simulink model "Tank_Modell_Student_2_tank_RL"  (R2020b)
settings: Solver=ode45  StartTime=0.0  StopTime=1200  RelTol=1e-3
values from neighbouring files (symbols this model uses):
  D = [0]    [Spielwiese.m]    (also in set_parameter.m; set_parameter_2_tank.m; set_parameter_3_tank.m)
undefined symbols (not defined in the file or in its folder): parRateLim, parReg, parSys
settings Model: Creator=Wolfgang Kemmetmüller  LastModifiedBy=simon
settings DataIOCC: LimitDataPoints=on  SaveFormat=Array  ReturnWorkspaceOutputs=off
settings OptimizationCC: BlockReduction=off  BooleanDataType=off  LifeSpan=inf
settings DebuggingCC: SaveWithParameterizedLinksMsg=none  UnderspecifiedInitializationDetection=Classic  MergeDetectMultiDrivingBlocksExec=none  SignalResolutionControl=TryResolveAllWithWarning  SFUnexpectedBacktrackingDiag=warning  SFNoUnconditionalDefaultTransitionDiag=warning  SFExecutionAtInitializationDiag=none  ArithmeticOperatorsInVariantConditions=warning
settings HardwareCC: ProdBitPerPointer=32  ProdBitPerSizeT=32  ProdBitPerPtrDiffT=32  ProdLargestAtomicFloat=None  ProdIntDivRoundTo=Undefined  ProdEndianess=Unspecified  ProdWordSize=32  ProdHWDeviceType=32-bit Generic  TargetUnknown=on
settings ModelReferenceCC: PropagateSignalLabelsOutOfModel=off
settings SFSimCC: SimUseLocalCustomCode=off  CustomCodeUndefinedFunction=UseInterfaceOnly
settings RTWCC: RTWUseLocalCustomCode=off
settings CodeAppCC: StateflowObjectComments=on
settings GRTTargetCC: TargetLangStandard=C89/C90 (ANSI)
settings ConfigComp: CovMetricSettings=dw  CovSaveCumulativeToWorkspaceVar=on  CovSaveSingleToWorkspaceVar=on  CovExternalEMLEnable=off

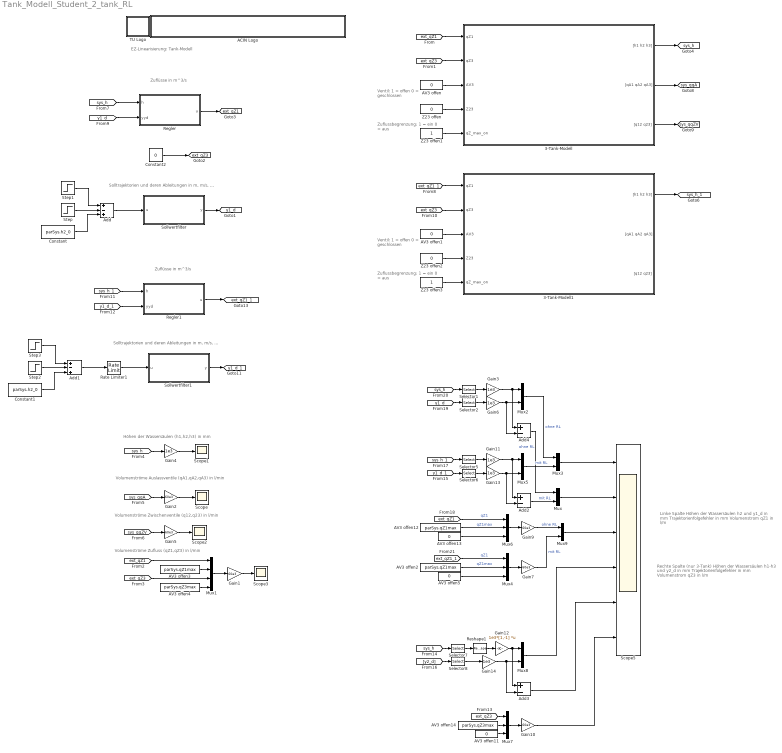
== system Tank_Modell_Student_2_tank_RL ==
  note: EZ-Linearisierung: Tank-Modell
  note: Höhen der Wassersäulen (h1,h2,h3) in mm
  note: Volumenströme Auslassventile (qA1,qA2,qA3) in l/min
  note: Volumenströme Zwischenventile (q12,q23) in l/min
  note: Ventil:
      | 1 = offen
      | 0 = geschlossen
  note: Volumenströme Zufluss (qZ1,qZ3) in l/min
  note: Linke Spalte
      | Höhen der Wassersäulen h2 und y1_d in mm
      | Trajektorienfolgefehler in mm
      | Volumenstrom qZ1 in l/m
  note: Zuflussbegrenzung:
      | 1 = ein
      | 0 = aus
  note: Rechte Spalte (nur 3-Tank)
      | Höhen der Wassersäulen h1-h3 und y2_d in mm
      | Trajektorienfolgefehler in mm
      | Volumenstrom qZ3 in l/m
  note: Zuflüsse in m^3/s
  note: Solltrajektorien und deren Ableitungen in m, m/s, ...
  note: Zuflussbegrenzung:
      | 1 = ein
      | 0 = aus
  note: Ventil:
      | 1 = offen
      | 0 = geschlossen
  note: Solltrajektorien und deren Ableitungen in m, m/s, ...
  note: Zuflüsse in m^3/s
  3-Tank-Modell : Subsystem
      mask init:
      | S = get_param(gcb,'UserData');
      mask Display:
      | image(S.pic);
      | port_label('input', 1, 'qZ1');
      | port_label('input', 2, 'qZ3');
      | port_label('input', 3, 'AV3');
      | port_label('input', 4, 'Z23');
      | port_label('input', 5, 'q_max_on');
      | port_label('output', 1, '[h1 h2 h3]');
      | port_label('output', 2, '[qA1 qA2 qA3]');
      | port_label('output', 3, '[q12 q23]');
  3-Tank-Modell1 : Subsystem
      mask init:
      | S = get_param(gcb,'UserData');
      mask Display:
      | image(S.pic);
      | port_label('input', 1, 'qZ1');
      | port_label('input', 2, 'qZ3');
      | port_label('input', 3, 'AV3');
      | port_label('input', 4, 'Z23');
      | port_label('input', 5, 'q_max_on');
      | port_label('output', 1, '[h1 h2 h3]');
      | port_label('output', 2, '[qA1 qA2 qA3]');
      | port_label('output', 3, '[q12 q23]');
  ACIN Logo : Subsystem
      mask init:
      | s = get_param(gcb,'UserData');
      mask Display:
      | image(s.logo,[0 0 439 45]);
      | %axis image
  AV3 offen{,1,5,11,13} (5 alike) : Constant  Value=0
  AV3 offen12 : Constant  Value=parSys.qZ1max  SampleTime=parSys.Ta
  AV3 offen14 : Constant  Value=parSys.qZ3max  SampleTime=parSys.Ta
  AV3 offen2 : Constant  Value=parSys.qZ1max  SampleTime=parSys.Ta
  AV3 offen3 : Constant  Value=parSys.qZ1max  SampleTime=parSys.Ta
  AV3 offen4 : Constant  Value=parSys.qZ3max  SampleTime=parSys.Ta
  Add : Sum  Inputs=+-+
  Add1 : Sum  Inputs=+-+
  Add2 : Sum  Inputs=+-
  Add3 : Sum  Inputs=+-
  Add4 : Sum  Inputs=+-
  Constant : Constant  Value=parSys.h2_0
  Constant1 : Constant  Value=parSys.h2_0
  Constant2 : Constant  Value=0
  Gain{1..2,5,7,9..10} (6 alike) : Gain  Gain=60e3
  Gain{3..4,6,11,13..14} (6 alike) : Gain  Gain=1e3
  Gain12 : Gain  Gain=1e3*[1,-1]  Multiplication=Matrix(K*u)
  Mux{,2..3,5,8..9} (6 alike) : Mux  Inputs=2
  Mux1 : Mux
  Mux4 : Mux  Inputs=3
  Mux6 : Mux  Inputs=3
  Mux7 : Mux  Inputs=3
  Rate Limiter1 : RateLimiter  RisingSlewLimit=parRateLim.delta_h_pos  FallingSlewLimit=parRateLim.delta_h_neg  SampleTimeMode=inherited
  Regler : MATLAB Function  TreatAsAtomicUnit=on
  Regler1 : MATLAB Function  TreatAsAtomicUnit=on
  Reshape1 : Reshape  OutputDimensionality=Column vector (2-D)
  Scope{,1..3} (4 alike) : Scope
  Scope5 : Scope  NumInputPorts=6
  Selector1 : Selector  InputPortWidth=3  IndexOptions=Index vector (dialog)  Indices=[2]  OutputSizes=1
  Selector2 : Selector  InputPortWidth=3  IndexOptions=Index vector (dialog)  Indices=[1]  OutputSizes=1
  Selector5 : Selector  InputPortWidth=3  IndexOptions=Index vector (dialog)  Indices=[2]  OutputSizes=1
  Selector6 : Selector  InputPortWidth=3  IndexOptions=Index vector (dialog)  Indices=[1]  OutputSizes=1
  Selector7 : Selector  InputPortWidth=3  IndexOptions=Index vector (dialog)  Indices=[1 3]  OutputSizes=1
  Selector8 : Selector  InputPortWidth=2  IndexOptions=Index vector (dialog)  Indices=[1]  OutputSizes=1
  Sollwertfilter : MATLAB Function  TreatAsAtomicUnit=on
  Sollwertfilter1 : MATLAB Function  TreatAsAtomicUnit=on
  Step : Step  Time=600  After=1*0.1  SampleTime=0
  Step1 : Step  Time=100  After=0.1  SampleTime=0
  Step2 : Step  Time=600  After=1*0.1  SampleTime=0
  Step3 : Step  Time=100  After=0.1  SampleTime=0
  TU Logo : Subsystem
      mask init:
      | s = get_param(gcb,'UserData');
      mask Display: image(s.logo,[0 0 45 45]);
  Z23 offen : Constant  Value=0
  Z23 offen1 : Constant
  Z23 offen2 : Constant  Value=0
  Z23 offen3 : Constant
  tag scope: ext_qZ1=global, ext_qZ1_1=global, ext_qZ3=global, sys_h=global, sys_h_1=global, sys_qqA=global, sys_qqZV=global, y1_d=global, y1_d_1=global
  wires:
  [sys_qqA] -> Gain2/1
  [sys_qqZV] -> Gain5/1
  [sys_h] -> Gain4/1
  3-Tank-Modell/1("[h1 h2 h3]") -> [sys_h]
  3-Tank-Modell/3("[q12 q23]") -> [sys_qqZV]
  3-Tank-Modell/2("[qA1 qA2 qA3]") -> [sys_qqA]
  AV3 offen/1 -> 3-Tank-Modell/3(AV3)
  Z23 offen/1 -> 3-Tank-Modell/4(Z23)
  [ext_qZ1] -> 3-Tank-Modell/1(qZ1)
  [ext_qZ3] -> 3-Tank-Modell/2(qZ3)
  [ext_qZ1] -> Mux1/1
  [ext_qZ3] -> Mux1/3
  AV3 offen3/1 -> Mux1/2
  AV3 offen4/1 -> Mux1/4
  Gain5/1 -> Scope2/1
  Gain2/1 -> Scope/1
  Gain4/1 -> Scope1/1
  Mux1/1 -> Gain1/1
  Gain1/1 -> Scope3/1
  Z23 offen1/1 -> 3-Tank-Modell/5(qZ_max_on)
  [ext_qZ3] -> Mux7/1
  Selector6/1 -> Gain13/1
  Mux7/1 -> Gain10/1
  AV3 offen11/1 -> Mux7/3
  [sys_h] -> Selector7/1
  AV3 offen14/1 -> Mux7/2
  [ext_qZ1] -> Mux6/1  "qZ1"
  Selector7/1 -> Reshape1/1
  Reshape1/1 -> Gain12/1
  [y2_d] -> Selector8/1
  Gain14/1 -> Mux8/2, Add3/2
  [sys_h_1] -> Selector5/1
  [y1_d_1] -> Selector6/1
  AV3 offen12/1 -> Mux6/2  "qZ1max"
  AV3 offen13/1 -> Mux6/3
  Selector8/1 -> Gain14/1
  Gain11/1 -> Add2/1, Mux5/1
  Add3/1 -> Scope5/5
  Mux6/1 -> Gain9/1
  Selector5/1 -> Gain11/1
  Gain13/1 -> Add2/2, Mux5/2
  Gain12/1 -> Mux8/1, Add3/1
  Gain10/1 -> Scope5/6
  Sollwertfilter/1(y) -> [y1_d]
  Step/1 -> Add/2
  Step1/1 -> Add/1
  Regler/1(u) -> [ext_qZ1]
  [sys_h] -> Regler/1(h)
  [y1_d] -> Regler/2(yyd)
  Constant/1 -> Add/3
  3-Tank-Modell1/1("[h1 h2 h3]") -> [sys_h_1]
  AV3 offen1/1 -> 3-Tank-Modell1/3(AV3)
  [ext_qZ1_1] -> 3-Tank-Modell1/1(qZ1)
  [ext_qZ3] -> 3-Tank-Modell1/2(qZ3)
  Z23 offen3/1 -> 3-Tank-Modell1/5(qZ_max_on)
  Z23 offen2/1 -> 3-Tank-Modell1/4(Z23)
  [y1_d_1] -> Regler1/2(yyd)
  [sys_h_1] -> Regler1/1(h)
  Sollwertfilter1/1(y) -> [y1_d_1]
  Constant1/1 -> Add1/3
  Step2/1 -> Add1/2
  Regler1/1(u) -> [ext_qZ1_1]
  Add1/1 -> Rate Limiter1/1
  Rate Limiter1/1 -> Sollwertfilter1/1(u)
  Step3/1 -> Add1/1
  Add/1 -> Sollwertfilter/1(u)
  Constant2/1 -> [ext_qZ3]
  Selector2/1 -> Gain6/1
  Gain3/1 -> Add4/1, Mux2/1
  [y1_d] -> Selector2/1
  [sys_h] -> Selector1/1
  Gain6/1 -> Add4/2, Mux2/2
  Selector1/1 -> Gain3/1
  Mux/1 -> Scope5/2
  Mux3/1 -> Scope5/1
  Mux2/1 -> Mux3/1  "ohne RL"
  Mux5/1 -> Mux3/2  "mit RL"
  Add4/1 -> Mux/1  "ohne RL"
  Add2/1 -> Mux/2  "mit RL"
  AV3 offen5/1 -> Mux4/3
  [ext_qZ1_1] -> Mux4/1  "qZ1"
  Mux4/1 -> Gain7/1
  AV3 offen2/1 -> Mux4/2  "qZ1max"
  Mux9/1 -> Scope5/3
  Gain9/1 -> Mux9/1  "ohne RL"
  Mux8/1 -> Scope5/4
  Gain7/1 -> Mux9/2  "mit RL"

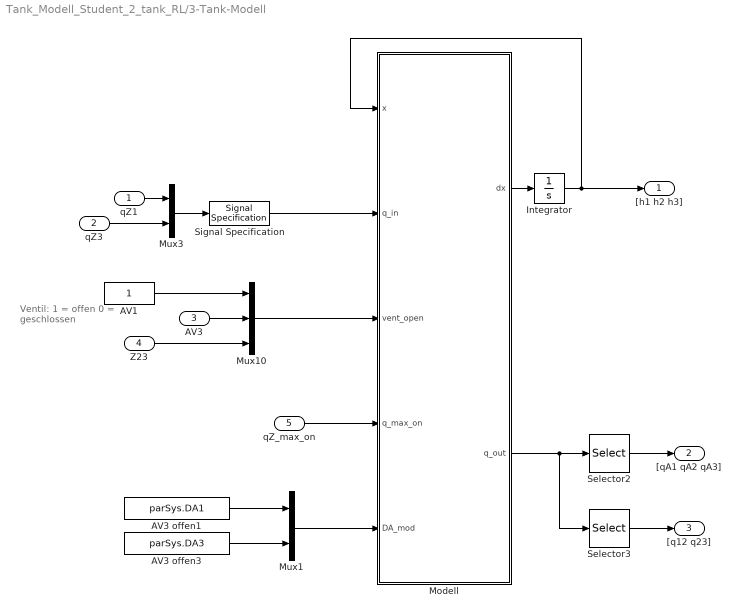
== system Tank_Modell_Student_2_tank_RL/3-Tank-Modell ==
  note: Ventil:
      | 1 = offen
      | 0 = geschlossen
  qZ1 : Inport
  qZ3 : Inport  Port=2
  AV3 : Inport  Port=3
  Z23 : Inport  Port=4
  qZ_max_on : Inport  Port=5
  AV1 : Constant
  AV3 offen1 : Constant  Value=parSys.DA1
  AV3 offen3 : Constant  Value=parSys.DA3
  Integrator : Integrator  InitialCondition=[parSys.h1_0;parSys.h2_0;parSys.h3_0]
  Modell : MATLAB Function  TreatAsAtomicUnit=on
  Mux1 : Mux  Inputs=2
  Mux10 : Mux  Inputs=3
  Mux3 : Mux  Inputs=2
  Selector2 : Selector  InputPortWidth=5  IndexOptions=Index vector (dialog)  Indices=[1 2 3]  OutputSizes=1
  Selector3 : Selector  InputPortWidth=5  IndexOptions=Index vector (dialog)  Indices=[4 5]  OutputSizes=1
  Signal Specification : SignalSpecification  Dimensions=2
  "[h1 h2 h3]" : Outport  VectorParamsAs1DForOutWhenUnconnected=off
  "[qA1 qA2 qA3]" : Outport  Port=2  VectorParamsAs1DForOutWhenUnconnected=off
  "[q12 q23]" : Outport  Port=3  VectorParamsAs1DForOutWhenUnconnected=off
  wires:
  AV1/1 -> Mux10/1
  qZ1/1 -> Mux3/1
  qZ3/1 -> Mux3/2
  Modell/2(q_out) -> Selector3/1, Selector2/1
  Selector2/1 -> "[qA1 qA2 qA3]"/1
  Selector3/1 -> "[q12 q23]"/1
  Z23/1 -> Mux10/3
  AV3/1 -> Mux10/2
  Mux10/1 -> Modell/3(vent_open)
  Mux3/1 -> Signal Specification/1
  Modell/1(dx) -> Integrator/1
  Integrator/1 -> Modell/1(x), "[h1 h2 h3]"/1
  Mux1/1 -> Modell/5(DA_mod)
  qZ_max_on/1 -> Modell/4(q_max_on)
  AV3 offen1/1 -> Mux1/1
  AV3 offen3/1 -> Mux1/2
  Signal Specification/1 -> Modell/2(q_in)

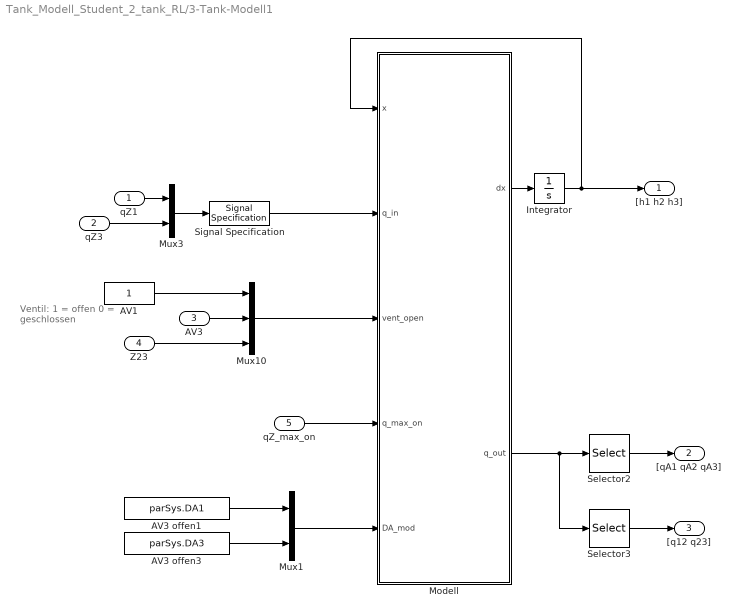
== system Tank_Modell_Student_2_tank_RL/3-Tank-Modell1 ==
  note: Ventil:
      | 1 = offen
      | 0 = geschlossen
  qZ1 : Inport
  qZ3 : Inport  Port=2
  AV3 : Inport  Port=3
  Z23 : Inport  Port=4
  qZ_max_on : Inport  Port=5
  AV1 : Constant
  AV3 offen1 : Constant  Value=parSys.DA1
  AV3 offen3 : Constant  Value=parSys.DA3
  Integrator : Integrator  InitialCondition=[parSys.h1_0;parSys.h2_0;parSys.h3_0]
  Modell : MATLAB Function  TreatAsAtomicUnit=on
  Mux1 : Mux  Inputs=2
  Mux10 : Mux  Inputs=3
  Mux3 : Mux  Inputs=2
  Selector2 : Selector  InputPortWidth=5  IndexOptions=Index vector (dialog)  Indices=[1 2 3]  OutputSizes=1
  Selector3 : Selector  InputPortWidth=5  IndexOptions=Index vector (dialog)  Indices=[4 5]  OutputSizes=1
  Signal Specification : SignalSpecification  Dimensions=2
  "[h1 h2 h3]" : Outport  VectorParamsAs1DForOutWhenUnconnected=off
  "[qA1 qA2 qA3]" : Outport  Port=2  VectorParamsAs1DForOutWhenUnconnected=off
  "[q12 q23]" : Outport  Port=3  VectorParamsAs1DForOutWhenUnconnected=off
  wires:
  AV1/1 -> Mux10/1
  qZ1/1 -> Mux3/1
  qZ3/1 -> Mux3/2
  Modell/2(q_out) -> Selector3/1, Selector2/1
  Selector2/1 -> "[qA1 qA2 qA3]"/1
  Selector3/1 -> "[q12 q23]"/1
  Z23/1 -> Mux10/3
  AV3/1 -> Mux10/2
  Mux10/1 -> Modell/3(vent_open)
  Mux3/1 -> Signal Specification/1
  Modell/1(dx) -> Integrator/1
  Integrator/1 -> Modell/1(x), "[h1 h2 h3]"/1
  Mux1/1 -> Modell/5(DA_mod)
  qZ_max_on/1 -> Modell/4(q_max_on)
  AV3 offen1/1 -> Mux1/1
  AV3 offen3/1 -> Mux1/2
  Signal Specification/1 -> Modell/2(q_in)

== system Tank_Modell_Student_2_tank_RL/ACIN Logo ==

== system Tank_Modell_Student_2_tank_RL/TU Logo ==

== matlab function Tank_Modell_Student_2_tank_RL/Regler ==
  settings: updateMethod=DISCRETE  sampleTime=0.2
  data: h input; yyd input; u output; parSys parameter; parReg parameter
function u = fcn(h,yyd,parSys,parReg)

% Parameter System
A_tank = parSys.Atank;
rho = parSys.rho;
eta = parSys.eta;
g = parSys.g;
alpha__A1 = parSys.alphaA1;
D__A1 = parSys.DA1;
alpha__A2 = parSys.alphaA2;
A__A2 = parSys.A2;
alpha__120 = parSys.alpha12_0;
A__12 = parSys.A12;
D__h12 = parSys.Dh12;
lambda__c12 = parSys.lambdac12;

% Parameter Regler
delta_h_min = parReg.delta_h_min;
a0 = parReg.a0;
a1 = parReg.a1;

% Sollwerte
yd = yyd(1);
ydp = yyd(2);
ydpp = yyd(3);

% Messgrößen
h1 = h(1);
h2 = h(2);

% Durchflüsse
qA1 = alpha__A1 * D__A1 ^ 2 * pi * sqrt(0.2e1) * sqrt(g * h1) / 0.4e1;
qA2 = alpha__A2 * A__A2 * sqrt(0.2e1) * sqrt(g * h2);
q12 = alpha__120 * tanh(0.2e1 * D__h12 * rho / eta * sqrt(0.2e1) * sqrt(g) * sqrt(abs(h1 - h2)) / lambda__c12) * A__12 * sqrt(0.2e1) * sqrt(g) * sqrt(abs(h1 - h2)) * sign((h1 - h2));

% Ableitungen der Durchflüsse
delta_h = h1-h2;
if(delta_h < delta_h_min)
    dq12_dh1 = -0.2e1 * delta_h_min ^ (-0.3e1 / 0.2e1) * A__12 * alpha__120 * (D__h12 * tanh(0.2e1 * D__h12 * rho / eta * sqrt(0.2e1) * sqrt(g) * sqrt(delta_h_min) / lambda__c12) ^ 2 * abs(delta_h) * sqrt(delta_h_min) * g * rho - tanh(0.2e1 * D__h12 * rho / eta * sqrt(0.2e1) * sqrt(g) * sqrt(delta_h_min) / lambda__c12) * abs(delta_h) * sqrt(0.2e1) * sqrt(g) * eta * lambda__c12 / 0.4e1 + g * rho * D__h12 * (abs(delta_h) * sqrt(delta_h_min) - 0.2e1 * delta_h_min ^ (0.3e1 / 0.2e1))) / eta / lambda__c12;
else
    dq12_dh1 = 0.2e1 * alpha__120 * D__h12 * rho / eta * g / lambda__c12 * (0.1e1 - tanh(0.2e1 * D__h12 * rho / eta * sqrt(0.2e1) * sqrt(g) * sqrt(abs(h1 - h2)) / lambda__c12) ^ 2) * A__12 + alpha__120 * tanh(0.2e1 * D__h12 * rho / eta * sqrt(0.2e1) * sqrt(g) * sqrt(abs(h1 - h2)) / lambda__c12) * A__12 * sqrt(0.2e1) * sqrt(g) * (abs(h1 - h2) ^ (-0.1e1 / 0.2e1)) / 0.2e1;
end
dq12_dh2 = -dq12_dh1;
dqA2_dh2 = alpha__A2 * A__A2 * sqrt(0.2e1) * (g * h2) ^ (-0.1e1 / 0.2e1) * g / 0.2e1;

% Lie Ableitungen
LgLf_h_ = 0.1e1 / A_tank ^ 2 * dq12_dh1;
LfLf_h_ = (dq12_dh1 * (-q12 - qA1) + (-dq12_dh2 + dqA2_dh2) * (qA2 - q12)) / A_tank ^ 2;
Lf_h_ = 0.1e1 / A_tank * (q12 - qA2);

% Stellgröße
u = 0.1e1 / LgLf_h_ * (ydpp - LfLf_h_ - a0 * (h2 - yd) - a1 * (Lf_h_ - ydp));
% if u < 0
%     u = 0;
% end

== matlab function Tank_Modell_Student_2_tank_RL/Sollwertfilter ==
  settings: updateMethod=DISCRETE  sampleTime=0.2
  data: u input; y output; parSollFilt parameter
function y = fcn(u,parSollFilt)
persistent x;
if isempty(x)
    x=[parSollFilt.yd0;0;0];
end
y = parSollFilt.C*x;
x = parSollFilt.A*x + parSollFilt.B*u;

== matlab function Tank_Modell_Student_2_tank_RL/3-Tank-Modell1/Modell ==
  data: dx output; x input; q_in input; vent_open input; q_max_on input; DA_mod input; q_out output; parSys parameter
function [dx,q_out] = fcn(x,q_in,vent_open,q_max_on,DA_mod,parSys)
%#codegen

[dx,q_out] = Wassertank_mfun(x,q_in,vent_open,q_max_on,DA_mod,parSys);


% Function end
end

== matlab function Tank_Modell_Student_2_tank_RL/Regler1 ==
  settings: updateMethod=DISCRETE  sampleTime=0.2
  data: h input; yyd input; u output; parSys parameter; parReg parameter
function u = fcn(h,yyd,parSys,parReg)

% Parameter System
A_tank = parSys.Atank;
rho = parSys.rho;
eta = parSys.eta;
g = parSys.g;
alpha__A1 = parSys.alphaA1;
D__A1 = parSys.DA1;
alpha__A2 = parSys.alphaA2;
A__A2 = parSys.A2;
alpha__120 = parSys.alpha12_0;
A__12 = parSys.A12;
D__h12 = parSys.Dh12;
lambda__c12 = parSys.lambdac12;

% Parameter Regler
delta_h_min = parReg.delta_h_min;
a0 = parReg.a0;
a1 = parReg.a1;

% Sollwerte
yd = yyd(1);
ydp = yyd(2);
ydpp = yyd(3);

% Messgrößen
h1 = h(1);
h2 = h(2);

% Durchflüsse
qA1 = alpha__A1 * D__A1 ^ 2 * pi * sqrt(0.2e1) * sqrt(g * h1) / 0.4e1;
qA2 = alpha__A2 * A__A2 * sqrt(0.2e1) * sqrt(g * h2);
q12 = alpha__120 * tanh(0.2e1 * D__h12 * rho / eta * sqrt(0.2e1) * sqrt(g) * sqrt(abs(h1 - h2)) / lambda__c12) * A__12 * sqrt(0.2e1) * sqrt(g) * sqrt(abs(h1 - h2)) * sign((h1 - h2));

% Ableitungen der Durchflüsse
delta_h = h1-h2;
if(delta_h < delta_h_min)
    dq12_dh1 = -0.2e1 * delta_h_min ^ (-0.3e1 / 0.2e1) * A__12 * alpha__120 * (D__h12 * tanh(0.2e1 * D__h12 * rho / eta * sqrt(0.2e1) * sqrt(g) * sqrt(delta_h_min) / lambda__c12) ^ 2 * abs(delta_h) * sqrt(delta_h_min) * g * rho - tanh(0.2e1 * D__h12 * rho / eta * sqrt(0.2e1) * sqrt(g) * sqrt(delta_h_min) / lambda__c12) * abs(delta_h) * sqrt(0.2e1) * sqrt(g) * eta * lambda__c12 / 0.4e1 + g * rho * D__h12 * (abs(delta_h) * sqrt(delta_h_min) - 0.2e1 * delta_h_min ^ (0.3e1 / 0.2e1))) / eta / lambda__c12;
else
    dq12_dh1 = 0.2e1 * alpha__120 * D__h12 * rho / eta * g / lambda__c12 * (0.1e1 - tanh(0.2e1 * D__h12 * rho / eta * sqrt(0.2e1) * sqrt(g) * sqrt(abs(h1 - h2)) / lambda__c12) ^ 2) * A__12 + alpha__120 * tanh(0.2e1 * D__h12 * rho / eta * sqrt(0.2e1) * sqrt(g) * sqrt(abs(h1 - h2)) / lambda__c12) * A__12 * sqrt(0.2e1) * sqrt(g) * (abs(h1 - h2) ^ (-0.1e1 / 0.2e1)) / 0.2e1;
end
dq12_dh2 = -dq12_dh1;
dqA2_dh2 = alpha__A2 * A__A2 * sqrt(0.2e1) * (g * h2) ^ (-0.1e1 / 0.2e1) * g / 0.2e1;

% Lie Ableitungen
LgLf_h_ = 0.1e1 / A_tank ^ 2 * dq12_dh1;
LfLf_h_ = (dq12_dh1 * (-q12 - qA1) + (-dq12_dh2 + dqA2_dh2) * (qA2 - q12)) / A_tank ^ 2;
Lf_h_ = 0.1e1 / A_tank * (q12 - qA2);

% Stellgröße
u = 0.1e1 / LgLf_h_ * (ydpp - LfLf_h_ - a0 * (h2 - yd) - a1 * (Lf_h_ - ydp));
% if u < 0
%     u = 0;
% end

== matlab function Tank_Modell_Student_2_tank_RL/3-Tank-Modell/Modell ==
  data: dx output; x input; q_in input; vent_open input; q_max_on input; DA_mod input; q_out output; parSys parameter
function [dx,q_out] = fcn(x,q_in,vent_open,q_max_on,DA_mod,parSys)
%#codegen

[dx,q_out] = Wassertank_mfun(x,q_in,vent_open,q_max_on,DA_mod,parSys);


% Function end
end

== matlab function Tank_Modell_Student_2_tank_RL/Sollwertfilter1 ==
  settings: updateMethod=DISCRETE  sampleTime=0.2
  data: u input; y output; parSollFilt_1 parameter
function y = fcn(u,parSollFilt_1)
persistent x;
if isempty(x)
    x=[parSollFilt_1.yd0;0;0];
end
y = parSollFilt_1.C*x;
x = parSollFilt_1.A*x + parSollFilt_1.B*u;
